simulink model "WF_onshore"  (R2024a)
settings: Solver=VariableStepAuto  StartTime=0  StopTime=0.9  RelTol=1e-3
values from neighbouring files (symbols this model uses):
  cvtr = initialize_NR_VSC_GF(cvtr)    [NR_steadystate_VSC_GF.m]    (also in WF_onshore_SSO_GFL.m = setfield(cvtr,'parameters', p_vary.name,p_vary.val(i)); WF_physical_param_offshore_supersynchronous.m = setfield(cvtr,'parameters', p_vary.name,p_vary.val(i)); WF_physical_param_onshore_SSO_020625.m = setfield(cvtr,'parameters', p_vary.name,p_vary.val(i)); impedance_WT_blackbox.m = base_values(cvtr))
  cvtr1 = cvtr_agg    [WF_physical_param_onshore_SSO_020625.m]
  enable_pll = 1    [impedance_WT_agg.m]    (also in initialize_WT_agg.m; initialize_WT_default_gfl.m; initialize_WT_default_offshore_super.m)
  f1 = 50    [WF_onshore_SSO_GFL.m]    (also in WF_physical_param_offshore_supersynchronous.m; WF_physical_param_onshore_SSO_020625.m; initialize_params_agg.m)
  i = 1    [WF_physical_param_offshore_supersynchronous.m]    (also in WF_physical_param_onshore_SSO_020625.m)
  L = inv(R)    [participation_factors_VSC_GF.m]
  l_OH = 0.2    [WF_onshore_SSO_GFL.m]    (also in WF_physical_param_offshore_supersynchronous.m = 0.1; WF_physical_param_onshore_SSO_020625.m = 0.1; initialize_params_agg.m = 0.1)
  l_tf_wf = tf_params(2,2)    [IM_WF_agg.m]    (also in WF_onshore_SSO_GFL.m = 0.05; WF_physical_param_offshore_supersynchronous.m = 0.05; WF_physical_param_onshore_SSO_020625.m = 0.05; initialize_params_agg.m = 0.05)
  l_tf_wt = tf_params(1,2)    [IM_WF_agg.m]    (also in WF_onshore_SSO_GFL.m = 0.0392; WF_physical_param_offshore_supersynchronous.m = 0.0392; WF_physical_param_onshore_SSO_020625.m = 0.0392; initialize_params_agg.m = 0.0392)
  Lg = p_vary(i)*((Z_b_G/(2*pi*f1)))    [WF_onshore_SSO_GFL.m]    (also in WF_physical_param_offshore_supersynchronous.m; WF_physical_param_onshore_SSO_020625.m; initialize_params_agg.m = 0.1*((Z_b_G/(2*pi*f1))))
  Lg1 = Lg    [WF_physical_param_offshore_supersynchronous.m]    (also in WF_physical_param_onshore_SSO_020625.m)
  Lg2 = Lg    [WF_physical_param_offshore_supersynchronous.m]    (also in WF_physical_param_onshore_SSO_020625.m)
  r_OH = 0.02    [WF_onshore_SSO_GFL.m]    (also in WF_physical_param_offshore_supersynchronous.m = 0.01; WF_physical_param_onshore_SSO_020625.m = 0.01; initialize_params_agg.m)
  r_tf_wf = tf_params(2,1)    [IM_WF_agg.m]    (also in WF_onshore_SSO_GFL.m = 0.005; WF_physical_param_offshore_supersynchronous.m = 0.005; WF_physical_param_onshore_SSO_020625.m = 0.005; initialize_params_agg.m = 0.005)
  r_tf_wt = tf_params(1,1)    [IM_WF_agg.m]    (also in WF_onshore_SSO_GFL.m = 0.0056; WF_physical_param_offshore_supersynchronous.m = 0.0056; WF_physical_param_onshore_SSO_020625.m = 0.0056; initialize_params_agg.m = 0.0056)
  Rg = rg*Z_b_G    [WF_onshore_SSO_GFL.m]    (also in WF_physical_param_offshore_supersynchronous.m; WF_physical_param_onshore_SSO_020625.m; initialize_params_agg.m = 0.01*Z_b_G)
  Sb_WF = (3*1)*5e6    (= 15000000)    [WF_onshore_SSO_GFL.m]    (also in WF_physical_param_offshore_supersynchronous.m; WF_physical_param_onshore_SSO_020625.m; impedance_WT_blackbox.m = n_t*Sb_WT; initialize_params_agg.m = 1000000000)
  Sb_WT = 5e6    (= 5000000)    [IM_WF.m]    (also in WF_onshore_SSO_GFL.m; WF_physical_param_offshore_supersynchronous.m; WF_physical_param_onshore_SSO_020625.m; initialize_params_agg.m)
  selector_current_reference = 3    [impedance_WT_agg.m]    (also in initialize_WT_agg.m; initialize_WT_default_gfl.m; initialize_WT_default_offshore_super.m)
  selector_omega_reference = 1    [impedance_WT_agg.m]    (also in initialize_WT_agg.m; initialize_WT_default_gfl.m; initialize_WT_default_offshore_super.m)
  V_coll = 33e3    (= 33000)    [WF_onshore_SSO_GFL.m]    (also in WF_physical_param_offshore_supersynchronous.m; WF_physical_param_onshore_SSO_020625.m; initialize_params_agg.m)
  V_trans = 220e3    (= 220000)    [WF_onshore_SSO_GFL.m]    (also in WF_physical_param_offshore_supersynchronous.m; WF_physical_param_onshore_SSO_020625.m; initialize_params_agg.m)
  Z_b_G = (V_trans/sqrt(3/2))^2/Sb_WF    [WF_onshore_SSO_GFL.m]    (also in WF_physical_param_offshore_supersynchronous.m = (V_b_trans)^2/Sb_WF; WF_physical_param_onshore_SSO_020625.m = (V_b_trans)^2/Sb_WF; initialize_params_agg.m = (V_b_trans)^2/Sb_WF)
undefined symbols (not defined in the file or in its folder): opts, R
libraries: simulink_extras x104, spsSeriesRLCBranchLib x90, simulink x52, spsThreePhaseVIMeasurementLib x42, spsControlledVoltageSourceLib x42, spsGroundLib x27, spsThreePhaseTransformerTwoWindingsLib x14, powerlib_extras x13, spsVariableInductorLib x6, spsPower3phInstantaneousLib x3, spspowerguiLib x1
(part 3 of 12)

== system WF_onshore/VoltageSource/grid inductance1 ==
  Rate Limiter : RateLimiter  SampleTimeMode=inherited
  Series RLC Branch : spsSeriesRLCBranchLib/Series RLC Branch  LConnTagsString=__new0  RConnTagsString=__new0  BranchType=R  Resistance=Rg+r_OH*Z_b_G  Inductance=Lg  SetiL0=off  InitialCurrent=cvtr.ss.io0a  Capacitance=1e-6  Setx0=off  InitialVoltage=0  Measurements=None
  Series RLC Branch1 : spsSeriesRLCBranchLib/Series RLC Branch  LConnTagsString=__new0  RConnTagsString=__new0  BranchType=R  Resistance=Rg+r_OH*Z_b_G  Inductance=Lg  SetiL0=off  InitialCurrent=cvtr.ss.io0b  Capacitance=1e-6  Setx0=off  InitialVoltage=0  Measurements=None
  Series RLC Branch2 : spsSeriesRLCBranchLib/Series RLC Branch  LConnTagsString=__new0  RConnTagsString=__new0  BranchType=R  Resistance=Rg+r_OH*Z_b_G  Inductance=Lg  SetiL0=off  InitialCurrent=cvtr.ss.io0c  Capacitance=1e-6  Setx0=off  InitialVoltage=0  Measurements=None
  Series RLC Branch3 : spsSeriesRLCBranchLib/Series RLC Branch  LConnTagsString=__new0  RConnTagsString=__new0  BranchType=R  Resistance=1e9  Inductance=Lg  SetiL0=off  InitialCurrent=cvtr.ss.io0a  Capacitance=1e-6  Setx0=off  InitialVoltage=0  Measurements=None
  Series RLC Branch4 : spsSeriesRLCBranchLib/Series RLC Branch  LConnTagsString=__new0  RConnTagsString=__new0  BranchType=R  Resistance=1e9  Inductance=Lg  SetiL0=off  InitialCurrent=cvtr.ss.io0a  Capacitance=1e-6  Setx0=off  InitialVoltage=0  Measurements=None
  Series RLC Branch5 : spsSeriesRLCBranchLib/Series RLC Branch  LConnTagsString=__new0  RConnTagsString=__new0  BranchType=R  Resistance=1e9  Inductance=Lg  SetiL0=off  InitialCurrent=cvtr.ss.io0a  Capacitance=1e-6  Setx0=off  InitialVoltage=0  Measurements=None
  Step : Step  Time=0.2  Before=(Lg1+l_OH*(Z_b_G/(2*pi*f1)))  After=(Lg2+l_OH*(Z_b_G/(2*pi*f1)))  SampleTime=0
  Variable Inductor : spsVariableInductorLib/Variable Inductor  methode=Backward Euler  Labsmin=1e-6  Initialize=off  iL0=0  L0=1e-3  Vl0=0
      settings: LibrarySourceBlock=sps_lib/Passives/Variable Inductor
  Variable Inductor1 : spsVariableInductorLib/Variable Inductor  methode=Backward Euler  Labsmin=1e-6  Initialize=off  iL0=0  L0=1e-3  Vl0=0
      settings: LibrarySourceBlock=sps_lib/Passives/Variable Inductor
  Variable Inductor2 : spsVariableInductorLib/Variable Inductor  methode=Backward Euler  Labsmin=1e-6  Initialize=off  iL0=0  L0=1e-3  Vl0=0
      settings: LibrarySourceBlock=sps_lib/Passives/Variable Inductor
  A : PMIOPort  Side=Left
  a : PMIOPort  Port=2  Side=Right
  B : PMIOPort  Port=3  Side=Left
  b : PMIOPort  Port=4  Side=Right
  C : PMIOPort  Port=5  Side=Left
  c : PMIOPort  Port=6  Side=Right
  wires:
  Step/1 -> Rate Limiter/1
  Rate Limiter/1 -> Variable Inductor2/1, Variable Inductor1/1, Variable Inductor/1
  connections:
  Series RLC Branch2/RConn1 -- c/RConn1
  Series RLC Branch1/RConn1 -- b/RConn1
  Series RLC Branch/RConn1 -- a/RConn1
  Series RLC Branch/LConn1 -- Series RLC Branch5/RConn1 -- Variable Inductor/RConn1
  Series RLC Branch1/LConn1 -- Series RLC Branch4/RConn1 -- Variable Inductor1/RConn1
  Series RLC Branch2/LConn1 -- Series RLC Branch3/RConn1 -- Variable Inductor2/RConn1
  A/RConn1 -- Series RLC Branch5/LConn1 -- Variable Inductor/LConn1
  B/RConn1 -- Series RLC Branch4/LConn1 -- Variable Inductor1/LConn1
  C/RConn1 -- Series RLC Branch3/LConn1 -- Variable Inductor2/LConn1

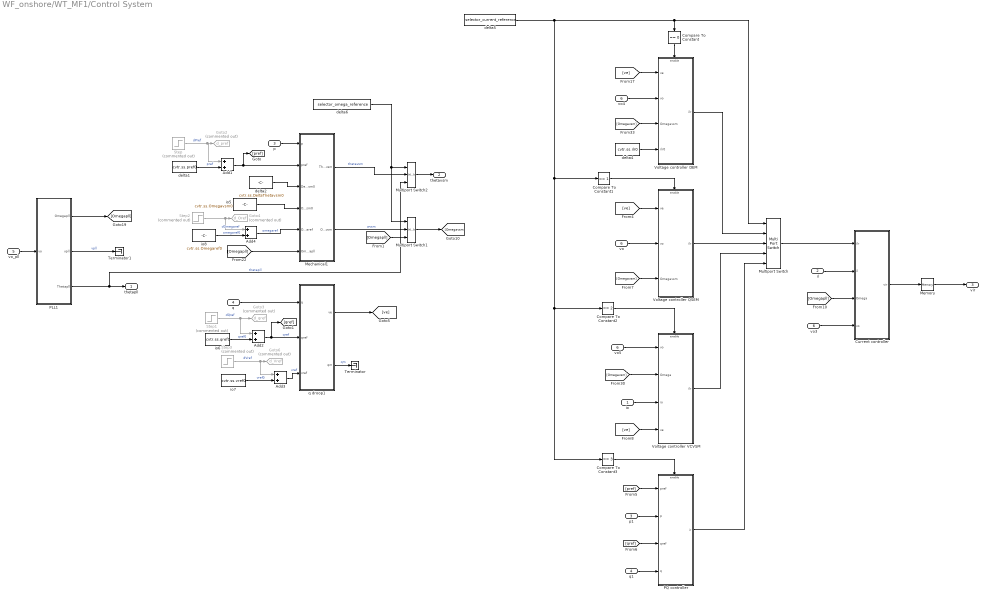
== system WF_onshore/WT_MF1/Control System ==
  io : Inport
  il : Inport  Port=2
  p : Inport  Port=3
  q : Inport  Port=4
  vo_pll : Inport  Port=5
  vo : Inport  Port=6
  Add{1..4} (4 alike) : Sum
  Compare To Constant : simulink/Logic and Bit Operations/Compare To Constant  relop===  const=0  OutDataTypeStr=boolean
  Compare To Constant1 : simulink/Logic and Bit Operations/Compare To Constant  relop===  const=1  OutDataTypeStr=boolean
  Compare To Constant2 : simulink/Logic and Bit Operations/Compare To Constant  relop===  const=2  OutDataTypeStr=boolean
  Compare To Constant3 : simulink/Logic and Bit Operations/Compare To Constant  relop===  const=3  OutDataTypeStr=boolean
  Current controller : Subsystem
  Goto2 : Goto  Commented=on  GotoTag=d_pref  TagVisibility=global
  Goto3 : Goto  Commented=on  GotoTag=d_qref  TagVisibility=global
  Goto4 : Goto  Commented=on  GotoTag=d_Oref  TagVisibility=global
  Goto6 : Goto  Commented=on  GotoTag=d_Vref  TagVisibility=global
  Mechanical1 : Subsystem
  Memory : Memory  InitialCondition=cvtr.ss.vir0
  Multiport Switch : MultiPortSwitch  DataPortOrder=Zero-based contiguous  Inputs=4  zeroidx=on  SaturateOnIntegerOverflow=off  InputSameDT=off
  Multiport Switch1 : MultiPortSwitch  DataPortOrder=Zero-based contiguous  Inputs=2  zeroidx=on  SaturateOnIntegerOverflow=off  InputSameDT=off
  Multiport Switch2 : MultiPortSwitch  DataPortOrder=Zero-based contiguous  Inputs=2  zeroidx=on  SaturateOnIntegerOverflow=off  InputSameDT=off
  PLL1 : Subsystem
  PQ controller : Subsystem
  Step : Step  Commented=on  After=0.01  SampleTime=0
  Step1 : Step  Commented=on  Time=1.5  After=0.03  SampleTime=0
  Step2 : Step  Commented=on  Time=2  After=0.001  SampleTime=0
  Step3 : Step  Commented=on  Time=2  After=0.001  SampleTime=0
  Terminator : Terminator
  Terminator1 : Terminator
  Voltage controller DEM : Subsystem
  Voltage controller QSEM : Subsystem
  Voltage controller VCVSM : Subsystem
  delta1 : Constant  Value=cvtr.ss.pref0
  delta2 : Constant  Value=cvtr.ss.DeltaThetavsm0
  delta4 : Constant  Value=cvtr.ss.ilr0
  delta5 : Constant  Value=selector_current_reference
  delta6 : Constant  Value=selector_omega_reference
  io5 : Constant  Value=cvtr.ss.Omegavsm0
  io6 : Constant  Value=cvtr.ss.qref0
  io7 : Constant  Value=cvtr.ss.vref0
  io8 : Constant  Value=cvtr.ss.Omegaref0
  p1 : InportShadow  Port=3
  q droop1 : Subsystem
  q1 : InportShadow  Port=4
  vo3 : InportShadow  Port=6
  vo4 : InportShadow  Port=6
  vo5 : InportShadow  Port=6
  thetapll : Outport
  thetavsm : Outport  Port=2
  vir : Outport  Port=3
  wires:
  io5/1 -> Mechanical1/4(Omegavsm0)
  Voltage controller DEM/1(ilr) -> Multiport Switch/2
  Add1/1 -> [pref], Mechanical1/2(pref)
  delta4/1 -> Voltage controller DEM/4(ilr0)
  Multiport Switch/1 -> Current controller/1(ilr)
  delta2/1 -> Mechanical1/3(DeltaThetavsm0)
  Add2/1 -> [qref], q droop1/2(qref)  "qref"
  delta1/1 -> Add1/2  "pref"
  q droop1/2(qm) -> Terminator/1  "qm"
  Add4/1 -> Mechanical1/5(Omegaref)  "omegaref"
  io7/1 -> Add3/2  "vref0"
  [Omegavsm] -> Voltage controller QSEM/3(Omegavsm)
  io8/1 -> Add4/2  "omegaref0"
  Step/1 -> Add1/1, Goto2/1  "dPref"
  [ve] -> Voltage controller QSEM/1(ve)
  delta5/1 -> Compare To Constant3/1, Compare To Constant2/1, Compare To Constant1/1, Multiport Switch/1, Compare To Constant/1
  io6/1 -> Add2/2  "qref0"
  Add3/1 -> q droop1/3(vref)  "vref"
  q/1 -> q droop1/1(q)
  [Omegavsm] -> Voltage controller VCVSM/2(Omega)
  [ve] -> Voltage controller DEM/1(ve)
  [Omegapll] -> Mechanical1/6(Omegapll)
  [Omegavsm] -> Voltage controller DEM/3(Omegavsm)
  p/1 -> Mechanical1/1(p)
  Voltage controller VCVSM/1(ilr) -> Multiport Switch/4
  vo/1 -> Voltage controller QSEM/2(vo)
  vo_pll/1 -> PLL1/1(vo)
  PLL1/2(vpll) -> Terminator1/1  "vpll"
  q droop1/1(ve) -> [ve]
  Voltage controller QSEM/1(ilr) -> Multiport Switch/3
  Memory/1 -> vir/1
  Current controller/1(vir) -> Memory/1
  p1/1 -> PQ controller/2(p)
  q1/1 -> PQ controller/4(q)
  PQ controller/1(ir) -> Multiport Switch/5
  il/1 -> Current controller/2(il)
  delta6/1 -> Multiport Switch2/1, Multiport Switch1/1
  [Omegapll] -> Current controller/3(Omega)
  Mechanical1/2(Omegavsm) -> Multiport Switch1/2  "wvsm"
  [Omegapll] -> Multiport Switch1/3
  Multiport Switch2/1 -> thetavsm/1
  Mechanical1/1(Thetavsm) -> Multiport Switch2/2  "thetavsm"
  Compare To Constant/1 -> Voltage controller DEM/Enable
  Compare To Constant1/1 -> Voltage controller QSEM/Enable
  Compare To Constant2/1 -> Voltage controller VCVSM/Enable
  Compare To Constant3/1 -> PQ controller/Enable
  Multiport Switch1/1 -> [Omegavsm]
  PLL1/1(Omegapll) -> [Omegapll]
  PLL1/3(Thetapll) -> Multiport Switch2/3, thetapll/1  "thetapll"
  io/1 -> Voltage controller VCVSM/3(io)
  vo3/1 -> Current controller/4(vo)
  vo4/1 -> Voltage controller DEM/2(vo)
  vo5/1 -> Voltage controller VCVSM/1(vo)
  [ve] -> Voltage controller VCVSM/4(ve)
  [pref] -> PQ controller/1(pref)
  [qref] -> PQ controller/3(qref)
  Step1/1 -> Goto3/1, Add2/1  "dQref"
  Step2/1 -> Add4/1, Goto4/1  "dOmegaref"
  Step3/1 -> Add3/1, Goto6/1  "dVref"

== system WF_onshore/WT_MF1/Inverse Park1 ==
  x_dq : Inport
  delta : Inport  Port=2
  Demux1 : Demux  Outputs=2
  Fcn : Fcn  Expr=cos(u(3))*u(1)-sin(u(3))*u(2)
  Fcn1 : Fcn  Expr=cos(u(3)-2/3*pi)*u(1)-sin(u(3)-2/3*pi)*u(2)
  Fcn2 : Fcn  Expr=cos(u(3)+2/3*pi)*u(1)-sin(u(3)+2/3*pi)*u(2)
  Mux : Mux  Inputs=3
  Mux1 : Mux  Inputs=3
  x_abc : Outport
  wires:
  Mux/1 -> Fcn1/1, Fcn2/1, Fcn/1
  Demux1/2 -> Mux/2
  Demux1/1 -> Mux/1
  Fcn/1 -> Mux1/1
  Fcn1/1 -> Mux1/2
  Fcn2/1 -> Mux1/3
  Mux1/1 -> x_abc/1
  x_dq/1 -> Demux1/1
  delta/1 -> Mux/3

== system WF_onshore/WT_MF1/Subsystem1 ==
  v_abc : Inport
  Controlled Voltage Source : spsControlledVoltageSourceLib/Controlled Voltage Source  Initialize=on  Source_Type=AC  Amplitude=0  Phase=0  Frequency=0  Measurements=None
  Controlled Voltage Source1 : spsControlledVoltageSourceLib/Controlled Voltage Source  Initialize=on  Source_Type=AC  Amplitude=0  Phase=0  Frequency=0  Measurements=None
  Controlled Voltage Source2 : spsControlledVoltageSourceLib/Controlled Voltage Source  Initialize=on  Source_Type=AC  Amplitude=0  Phase=0  Frequency=0  Measurements=None
  Demux : Demux  Outputs=3
  Ground : spsGroundLib/Ground  LConnTagsString=a
  va1 : PMIOPort  Side=Right
  vb1 : PMIOPort  Port=2  Side=Right
  vc1 : PMIOPort  Port=3  Side=Right
  wires:
  v_abc/1 -> Demux/1
  Demux/3 -> Controlled Voltage Source2/1
  Demux/2 -> Controlled Voltage Source1/1
  Demux/1 -> Controlled Voltage Source/1
  connections:
  Controlled Voltage Source/LConn1 -- Controlled Voltage Source1/LConn1 -- Controlled Voltage Source2/LConn1 -- Ground/LConn1
  vc1/RConn1 -- Controlled Voltage Source2/RConn1
  vb1/RConn1 -- Controlled Voltage Source1/RConn1
  va1/RConn1 -- Controlled Voltage Source/RConn1

== system WF_onshore/WT_MF1/Subsystem6 ==
  x_d+ix_q : Inport
  Complex to Real-Imag2 : ComplexToRealImag
  Mux : Mux  Inputs=2
  x_dq : Outport
  wires:
  Complex to Real-Imag2/1 -> Mux/1
  Complex to Real-Imag2/2 -> Mux/2
  Mux/1 -> x_dq/1
  x_d+ix_q/1 -> Complex to Real-Imag2/1

== system WF_onshore/WT_MF1/Transformations (pu and dq) ==
  i_abc_grid : Inport
  i_abc_filt : Inport  Port=2
  v_abc_grid : Inport  Port=3
  v_abc_filt : Inport  Port=4
  Thetavsm : Inport  Port=5
  Thetapll : Inport  Port=6
  3-phase Instantaneous Active & Reactive Power : powerlib_extras/Measurements/3-phase  Instantaneous  Active & Reactive Power
  Demux : Demux  Outputs=2
  Gain : Gain  Gain=1/cvtr.pu.Vb
  Gain1 : Gain  Gain=1/cvtr.pu.Ib
  Gain2 : Gain  Gain=1/cvtr.pu.Sb
  Gain4 : Gain  Gain=1/cvtr.pu.Ib
  Gain6 : Gain  Gain=1/cvtr.pu.Vb
  I_conv : ToWorkspace  VariableName=I_dq  SaveFormat=Structure With Time  SampleTime=-1
      settings: MaxDataPoints=1000000
  Park : Subsystem
  Park1 : Subsystem
  Park2 : Subsystem
  Park4 : Subsystem
  Scope{,1..2,4} (4 alike) : Scope  Commented=on
  Scope3 : Scope  Commented=on  NumInputPorts=2
  Subsystem2 : Subsystem
  Subsystem3 : Subsystem
  Subsystem4 : Subsystem
  Subsystem7 : Subsystem
  V_conv : ToWorkspace  VariableName=V_dq  SaveFormat=Structure With Time  SampleTime=-1
      settings: MaxDataPoints=1000000
  io : Outport
  il : Outport  Port=2
  p : Outport  Port=3
  q : Outport  Port=4
  vo_pll : Outport  Port=5
  vo : Outport  Port=6
  wires:
  Gain6/1 -> Park4/1(x_abc)
  i_abc_grid/1 -> 3-phase Instantaneous Active & Reactive Power/2, Gain1/1
  Gain2/1 -> Demux/1
  Gain1/1 -> Park1/1(x_abc)
  Gain/1 -> Park2/1(x_abc)
  Gain4/1 -> Park/1(x_abc)
  Park4/1(x_dq) -> Subsystem2/1(x_dq)
  Demux/1 -> Scope3/1, p/1
  i_abc_filt/1 -> Gain4/1
  Thetapll/1 -> Park4/2(delta)
  Subsystem2/1(x_d+ix_q) -> Scope4/1, vo_pll/1
  Thetavsm/1 -> Park1/2(delta), Park2/2(delta), Park/2(delta)
  Demux/2 -> Scope3/2, q/1
  v_abc_grid/1 -> 3-phase Instantaneous Active & Reactive Power/1
  3-phase Instantaneous Active & Reactive Power/1 -> Gain2/1
  Subsystem4/1(x_d+ix_q) -> io/1
  Subsystem7/1(x_d+ix_q) -> il/1, Scope/1
  Subsystem3/1(x_d+ix_q) -> vo/1
  Park/1(x_dq) -> Subsystem7/1(x_dq)
  Park1/1(x_dq) -> I_conv/1, Scope2/1, Subsystem4/1(x_dq)
  Park2/1(x_dq) -> V_conv/1, Scope1/1, Subsystem3/1(x_dq)
  v_abc_filt/1 -> Gain/1, Gain6/1

== system WF_onshore/WT_MF1/filter capacitance1 ==
  Ground : spsGroundLib/Ground  LConnTagsString=a
  Series RLC Branch : spsSeriesRLCBranchLib/Series RLC Branch  LConnTagsString=__new0  RConnTagsString=__new0  BranchType=C  Resistance=R  Inductance=L  SetiL0=on  InitialCurrent=ia0  Capacitance=cvtr.parameters.Cf  Setx0=on  InitialVoltage=cvtr.ss.vo0a  Measurements=None
  Series RLC Branch1 : spsSeriesRLCBranchLib/Series RLC Branch  LConnTagsString=__new0  RConnTagsString=__new0  BranchType=C  Resistance=R  Inductance=L  SetiL0=on  InitialCurrent=ia0  Capacitance=cvtr.parameters.Cf  Setx0=on  InitialVoltage=cvtr.ss.vo0b  Measurements=None
  Series RLC Branch2 : spsSeriesRLCBranchLib/Series RLC Branch  LConnTagsString=__new0  RConnTagsString=__new0  BranchType=C  Resistance=R  Inductance=L  SetiL0=on  InitialCurrent=ia0  Capacitance=cvtr.parameters.Cf  Setx0=on  InitialVoltage=cvtr.ss.vo0c  Measurements=None
  Three-Phase V-I Measurement : spsThreePhaseVIMeasurementLib/Three-Phase V-I Measurement  VoltageMeasurement=phase-to-ground  SetLabelV=off  LabelV=Vabc  Vpu=off  VpuLL=off  CurrentMeasurement=no  SetLabelI=off  LabelI=Iabc  Ipu=off  Pbase=100e6  Vbase=500e3  OutputType=Complex  PhasorSimulation=off  PSBequivalent=0
  A : PMIOPort  Side=Left
  B : PMIOPort  Port=2  Side=Left
  C : PMIOPort  Port=3  Side=Left
  v_abc : Outport
  wires:
  Three-Phase V-I Measurement/1 -> v_abc/1
  connections:
  A/RConn1 -- Three-Phase V-I Measurement/LConn1
  B/RConn1 -- Three-Phase V-I Measurement/LConn2
  C/RConn1 -- Three-Phase V-I Measurement/LConn3
  Three-Phase V-I Measurement/RConn1 -- Series RLC Branch/LConn1
  Three-Phase V-I Measurement/RConn2 -- Series RLC Branch1/LConn1
  Three-Phase V-I Measurement/RConn3 -- Series RLC Branch2/LConn1
  Series RLC Branch/RConn1 -- Ground/LConn1 -- Series RLC Branch1/RConn1 -- Series RLC Branch2/RConn1

== system WF_onshore/WT_MF1/filter inductance1 ==
  Series RLC Branch : spsSeriesRLCBranchLib/Series RLC Branch  LConnTagsString=__new0  RConnTagsString=__new0  BranchType=RL  Resistance=cvtr.parameters.Rf  Inductance=cvtr.parameters.Lf  SetiL0=on  InitialCurrent=cvtr.ss.il0a  Capacitance=1e-6  Setx0=off  InitialVoltage=0  Measurements=None
  Series RLC Branch1 : spsSeriesRLCBranchLib/Series RLC Branch  LConnTagsString=__new0  RConnTagsString=__new0  BranchType=RL  Resistance=cvtr.parameters.Rf  Inductance=cvtr.parameters.Lf  SetiL0=on  InitialCurrent=cvtr.ss.il0b  Capacitance=1e-6  Setx0=off  InitialVoltage=0  Measurements=None
  Series RLC Branch2 : spsSeriesRLCBranchLib/Series RLC Branch  LConnTagsString=__new0  RConnTagsString=__new0  BranchType=RL  Resistance=cvtr.parameters.Rf  Inductance=cvtr.parameters.Lf  SetiL0=on  InitialCurrent=cvtr.ss.il0c  Capacitance=1e-6  Setx0=off  InitialVoltage=0  Measurements=None
  Three-Phase V-I Measurement : spsThreePhaseVIMeasurementLib/Three-Phase V-I Measurement  VoltageMeasurement=no  SetLabelV=off  LabelV=Vabc  Vpu=off  VpuLL=off  CurrentMeasurement=yes  SetLabelI=off  LabelI=Iabc  Ipu=off  Pbase=100e6  Vbase=500e3  OutputType=Complex  PhasorSimulation=off  PSBequivalent=0
  A : PMIOPort  Side=Left
  B : PMIOPort  Port=2  Side=Left
  C : PMIOPort  Port=3  Side=Left
  a : PMIOPort  Port=4  Side=Right
  b : PMIOPort  Port=5  Side=Right
  c : PMIOPort  Port=6  Side=Right
  i_abc : Outport
  wires:
  Three-Phase V-I Measurement/1 -> i_abc/1
  connections:
  c/RConn1 -- Three-Phase V-I Measurement/RConn3
  C/RConn1 -- Series RLC Branch2/LConn1
  b/RConn1 -- Three-Phase V-I Measurement/RConn2
  B/RConn1 -- Series RLC Branch1/LConn1
  a/RConn1 -- Three-Phase V-I Measurement/RConn1
  A/RConn1 -- Series RLC Branch/LConn1
  Series RLC Branch2/RConn1 -- Three-Phase V-I Measurement/LConn3
  Series RLC Branch1/RConn1 -- Three-Phase V-I Measurement/LConn2
  Series RLC Branch/RConn1 -- Three-Phase V-I Measurement/LConn1

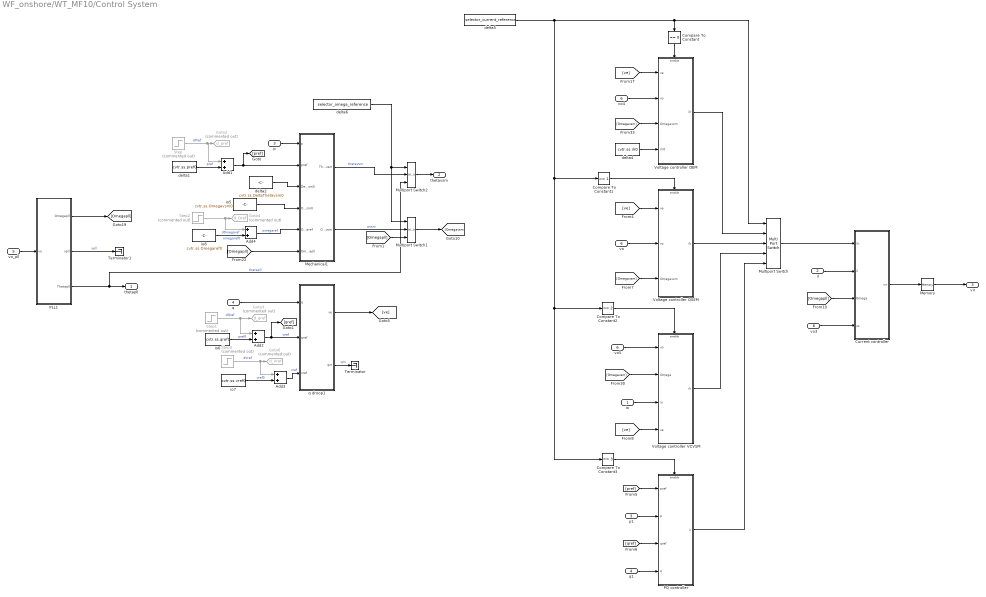
== system WF_onshore/WT_MF10/Control System ==
  io : Inport
  il : Inport  Port=2
  p : Inport  Port=3
  q : Inport  Port=4
  vo_pll : Inport  Port=5
  vo : Inport  Port=6
  Add{1..4} (4 alike) : Sum
  Compare To Constant : simulink/Logic and Bit Operations/Compare To Constant  relop===  const=0  OutDataTypeStr=boolean
  Compare To Constant1 : simulink/Logic and Bit Operations/Compare To Constant  relop===  const=1  OutDataTypeStr=boolean
  Compare To Constant2 : simulink/Logic and Bit Operations/Compare To Constant  relop===  const=2  OutDataTypeStr=boolean
  Compare To Constant3 : simulink/Logic and Bit Operations/Compare To Constant  relop===  const=3  OutDataTypeStr=boolean
  Current controller : Subsystem
  Goto2 : Goto  Commented=on  GotoTag=d_pref  TagVisibility=global
  Goto3 : Goto  Commented=on  GotoTag=d_qref  TagVisibility=global
  Goto4 : Goto  Commented=on  GotoTag=d_Oref  TagVisibility=global
  Goto6 : Goto  Commented=on  GotoTag=d_Vref  TagVisibility=global
  Mechanical1 : Subsystem
  Memory : Memory  InitialCondition=cvtr.ss.vir0
  Multiport Switch : MultiPortSwitch  DataPortOrder=Zero-based contiguous  Inputs=4  zeroidx=on  SaturateOnIntegerOverflow=off  InputSameDT=off
  Multiport Switch1 : MultiPortSwitch  DataPortOrder=Zero-based contiguous  Inputs=2  zeroidx=on  SaturateOnIntegerOverflow=off  InputSameDT=off
  Multiport Switch2 : MultiPortSwitch  DataPortOrder=Zero-based contiguous  Inputs=2  zeroidx=on  SaturateOnIntegerOverflow=off  InputSameDT=off
  PLL1 : Subsystem
  PQ controller : Subsystem
  Step : Step  Commented=on  After=0.01  SampleTime=0
  Step1 : Step  Commented=on  Time=1.5  After=0.03  SampleTime=0
  Step2 : Step  Commented=on  Time=2  After=0.001  SampleTime=0
  Step3 : Step  Commented=on  Time=2  After=0.001  SampleTime=0
  Terminator : Terminator
  Terminator1 : Terminator
  Voltage controller DEM : Subsystem
  Voltage controller QSEM : Subsystem
  Voltage controller VCVSM : Subsystem
  delta1 : Constant  Value=cvtr.ss.pref0
  delta2 : Constant  Value=cvtr.ss.DeltaThetavsm0
  delta4 : Constant  Value=cvtr.ss.ilr0
  delta5 : Constant  Value=selector_current_reference
  delta6 : Constant  Value=selector_omega_reference
  io5 : Constant  Value=cvtr.ss.Omegavsm0
  io6 : Constant  Value=cvtr.ss.qref0
  io7 : Constant  Value=cvtr.ss.vref0
  io8 : Constant  Value=cvtr.ss.Omegaref0
  p1 : InportShadow  Port=3
  q droop1 : Subsystem
  q1 : InportShadow  Port=4
  vo3 : InportShadow  Port=6
  vo4 : InportShadow  Port=6
  vo5 : InportShadow  Port=6
  thetapll : Outport
  thetavsm : Outport  Port=2
  vir : Outport  Port=3
  wires:
  Step3/1 -> Goto6/1, Add3/1  "dVref"
  Step2/1 -> Goto4/1, Add4/1  "dOmegaref"
  Step1/1 -> Add2/1, Goto3/1  "dQref"
  [qref] -> PQ controller/3(qref)
  [pref] -> PQ controller/1(pref)
  [ve] -> Voltage controller VCVSM/4(ve)
  vo5/1 -> Voltage controller VCVSM/1(vo)
  vo4/1 -> Voltage controller DEM/2(vo)
  vo3/1 -> Current controller/4(vo)
  io/1 -> Voltage controller VCVSM/3(io)
  PLL1/3(Thetapll) -> thetapll/1, Multiport Switch2/3  "thetapll"
  PLL1/1(Omegapll) -> [Omegapll]
  Multiport Switch1/1 -> [Omegavsm]
  Compare To Constant3/1 -> PQ controller/Enable
  Compare To Constant2/1 -> Voltage controller VCVSM/Enable
  Compare To Constant1/1 -> Voltage controller QSEM/Enable
  Compare To Constant/1 -> Voltage controller DEM/Enable
  Mechanical1/1(Thetavsm) -> Multiport Switch2/2  "thetavsm"
  Multiport Switch2/1 -> thetavsm/1
  [Omegapll] -> Multiport Switch1/3
  Mechanical1/2(Omegavsm) -> Multiport Switch1/2  "wvsm"
  [Omegapll] -> Current controller/3(Omega)
  delta6/1 -> Multiport Switch1/1, Multiport Switch2/1
  il/1 -> Current controller/2(il)
  PQ controller/1(ir) -> Multiport Switch/5
  q1/1 -> PQ controller/4(q)
  p1/1 -> PQ controller/2(p)
  Current controller/1(vir) -> Memory/1
  Memory/1 -> vir/1
  Voltage controller QSEM/1(ilr) -> Multiport Switch/3
  q droop1/1(ve) -> [ve]
  PLL1/2(vpll) -> Terminator1/1  "vpll"
  vo_pll/1 -> PLL1/1(vo)
  vo/1 -> Voltage controller QSEM/2(vo)
  Voltage controller VCVSM/1(ilr) -> Multiport Switch/4
  p/1 -> Mechanical1/1(p)
  [Omegavsm] -> Voltage controller DEM/3(Omegavsm)
  [Omegapll] -> Mechanical1/6(Omegapll)
  [ve] -> Voltage controller DEM/1(ve)
  [Omegavsm] -> Voltage controller VCVSM/2(Omega)
  q/1 -> q droop1/1(q)
  Add3/1 -> q droop1/3(vref)  "vref"
  io6/1 -> Add2/2  "qref0"
  delta5/1 -> Compare To Constant/1, Multiport Switch/1, Compare To Constant1/1, Compare To Constant2/1, Compare To Constant3/1
  [ve] -> Voltage controller QSEM/1(ve)
  Step/1 -> Goto2/1, Add1/1  "dPref"
  io8/1 -> Add4/2  "omegaref0"
  [Omegavsm] -> Voltage controller QSEM/3(Omegavsm)
  io7/1 -> Add3/2  "vref0"
  Add4/1 -> Mechanical1/5(Omegaref)  "omegaref"
  q droop1/2(qm) -> Terminator/1  "qm"
  delta1/1 -> Add1/2  "pref"
  Add2/1 -> q droop1/2(qref), [qref]  "qref"
  delta2/1 -> Mechanical1/3(DeltaThetavsm0)
  Multiport Switch/1 -> Current controller/1(ilr)
  delta4/1 -> Voltage controller DEM/4(ilr0)
  Add1/1 -> Mechanical1/2(pref), [pref]
  Voltage controller DEM/1(ilr) -> Multiport Switch/2
  io5/1 -> Mechanical1/4(Omegavsm0)

== system WF_onshore/WT_MF10/Inverse Park1 ==
  x_dq : Inport
  delta : Inport  Port=2
  Demux1 : Demux  Outputs=2
  Fcn : Fcn  Expr=cos(u(3))*u(1)-sin(u(3))*u(2)
  Fcn1 : Fcn  Expr=cos(u(3)-2/3*pi)*u(1)-sin(u(3)-2/3*pi)*u(2)
  Fcn2 : Fcn  Expr=cos(u(3)+2/3*pi)*u(1)-sin(u(3)+2/3*pi)*u(2)
  Mux : Mux  Inputs=3
  Mux1 : Mux  Inputs=3
  x_abc : Outport
  wires:
  delta/1 -> Mux/3
  x_dq/1 -> Demux1/1
  Mux1/1 -> x_abc/1
  Fcn2/1 -> Mux1/3
  Fcn1/1 -> Mux1/2
  Fcn/1 -> Mux1/1
  Demux1/1 -> Mux/1
  Demux1/2 -> Mux/2
  Mux/1 -> Fcn/1, Fcn2/1, Fcn1/1

== system WF_onshore/WT_MF10/Subsystem1 ==
  v_abc : Inport
  Controlled Voltage Source : spsControlledVoltageSourceLib/Controlled Voltage Source  Initialize=on  Source_Type=AC  Amplitude=0  Phase=0  Frequency=0  Measurements=None
  Controlled Voltage Source1 : spsControlledVoltageSourceLib/Controlled Voltage Source  Initialize=on  Source_Type=AC  Amplitude=0  Phase=0  Frequency=0  Measurements=None
  Controlled Voltage Source2 : spsControlledVoltageSourceLib/Controlled Voltage Source  Initialize=on  Source_Type=AC  Amplitude=0  Phase=0  Frequency=0  Measurements=None
  Demux : Demux  Outputs=3
  Ground : spsGroundLib/Ground  LConnTagsString=a
  va1 : PMIOPort  Side=Right
  vb1 : PMIOPort  Port=2  Side=Right
  vc1 : PMIOPort  Port=3  Side=Right
  wires:
  Demux/1 -> Controlled Voltage Source/1
  Demux/2 -> Controlled Voltage Source1/1
  Demux/3 -> Controlled Voltage Source2/1
  v_abc/1 -> Demux/1
  connections:
  va1/RConn1 -- Controlled Voltage Source/RConn1
  vb1/RConn1 -- Controlled Voltage Source1/RConn1
  vc1/RConn1 -- Controlled Voltage Source2/RConn1
  Ground/LConn1 -- Controlled Voltage Source2/LConn1 -- Controlled Voltage Source1/LConn1 -- Controlled Voltage Source/LConn1

== system WF_onshore/WT_MF10/Subsystem6 ==
  x_d+ix_q : Inport
  Complex to Real-Imag2 : ComplexToRealImag
  Mux : Mux  Inputs=2
  x_dq : Outport
  wires:
  x_d+ix_q/1 -> Complex to Real-Imag2/1
  Mux/1 -> x_dq/1
  Complex to Real-Imag2/2 -> Mux/2
  Complex to Real-Imag2/1 -> Mux/1

== system WF_onshore/WT_MF10/Transformations (pu and dq) ==
  i_abc_grid : Inport
  i_abc_filt : Inport  Port=2
  v_abc_grid : Inport  Port=3
  v_abc_filt : Inport  Port=4
  Thetavsm : Inport  Port=5
  Thetapll : Inport  Port=6
  3-phase Instantaneous Active & Reactive Power : powerlib_extras/Measurements/3-phase  Instantaneous  Active & Reactive Power
  Demux : Demux  Outputs=2
  Gain : Gain  Gain=1/cvtr.pu.Vb
  Gain1 : Gain  Gain=1/cvtr.pu.Ib
  Gain2 : Gain  Gain=1/cvtr.pu.Sb
  Gain4 : Gain  Gain=1/cvtr.pu.Ib
  Gain6 : Gain  Gain=1/cvtr.pu.Vb
  Park : Subsystem
  Park1 : Subsystem
  Park2 : Subsystem
  Park4 : Subsystem
  Subsystem2 : Subsystem
  Subsystem3 : Subsystem
  Subsystem4 : Subsystem
  Subsystem7 : Subsystem
  io : Outport
  il : Outport  Port=2
  p : Outport  Port=3
  q : Outport  Port=4
  vo_pll : Outport  Port=5
  vo : Outport  Port=6
  wires:
  v_abc_filt/1 -> Gain6/1, Gain/1
  Park2/1(x_dq) -> Subsystem3/1(x_dq)
  Park1/1(x_dq) -> Subsystem4/1(x_dq)
  Park/1(x_dq) -> Subsystem7/1(x_dq)
  Subsystem3/1(x_d+ix_q) -> vo/1
  Subsystem7/1(x_d+ix_q) -> il/1
  Subsystem4/1(x_d+ix_q) -> io/1
  3-phase Instantaneous Active & Reactive Power/1 -> Gain2/1
  v_abc_grid/1 -> 3-phase Instantaneous Active & Reactive Power/1
  Demux/2 -> q/1
  Thetavsm/1 -> Park/2(delta), Park2/2(delta), Park1/2(delta)
  Subsystem2/1(x_d+ix_q) -> vo_pll/1
  Thetapll/1 -> Park4/2(delta)
  i_abc_filt/1 -> Gain4/1
  Demux/1 -> p/1
  Park4/1(x_dq) -> Subsystem2/1(x_dq)
  Gain4/1 -> Park/1(x_abc)
  Gain/1 -> Park2/1(x_abc)
  Gain1/1 -> Park1/1(x_abc)
  Gain2/1 -> Demux/1
  i_abc_grid/1 -> Gain1/1, 3-phase Instantaneous Active & Reactive Power/2
  Gain6/1 -> Park4/1(x_abc)

== system WF_onshore/WT_MF10/filter capacitance1 ==
  Ground : spsGroundLib/Ground  LConnTagsString=a
  Series RLC Branch : spsSeriesRLCBranchLib/Series RLC Branch  LConnTagsString=__new0  RConnTagsString=__new0  BranchType=C  Resistance=R  Inductance=L  SetiL0=on  InitialCurrent=ia0  Capacitance=cvtr.parameters.Cf  Setx0=on  InitialVoltage=cvtr.ss.vo0a  Measurements=None
  Series RLC Branch1 : spsSeriesRLCBranchLib/Series RLC Branch  LConnTagsString=__new0  RConnTagsString=__new0  BranchType=C  Resistance=R  Inductance=L  SetiL0=on  InitialCurrent=ia0  Capacitance=cvtr.parameters.Cf  Setx0=on  InitialVoltage=cvtr.ss.vo0b  Measurements=None
  Series RLC Branch2 : spsSeriesRLCBranchLib/Series RLC Branch  LConnTagsString=__new0  RConnTagsString=__new0  BranchType=C  Resistance=R  Inductance=L  SetiL0=on  InitialCurrent=ia0  Capacitance=cvtr.parameters.Cf  Setx0=on  InitialVoltage=cvtr.ss.vo0c  Measurements=None
  Three-Phase V-I Measurement : spsThreePhaseVIMeasurementLib/Three-Phase V-I Measurement  VoltageMeasurement=phase-to-ground  SetLabelV=off  LabelV=Vabc  Vpu=off  VpuLL=off  CurrentMeasurement=no  SetLabelI=off  LabelI=Iabc  Ipu=off  Pbase=100e6  Vbase=500e3  OutputType=Complex  PhasorSimulation=off  PSBequivalent=0
  A : PMIOPort  Side=Left
  B : PMIOPort  Port=2  Side=Left
  C : PMIOPort  Port=3  Side=Left
  v_abc : Outport
  wires:
  Three-Phase V-I Measurement/1 -> v_abc/1
  connections:
  Series RLC Branch2/RConn1 -- Series RLC Branch1/RConn1 -- Ground/LConn1 -- Series RLC Branch/RConn1
  Three-Phase V-I Measurement/RConn3 -- Series RLC Branch2/LConn1
  Three-Phase V-I Measurement/RConn2 -- Series RLC Branch1/LConn1
  Three-Phase V-I Measurement/RConn1 -- Series RLC Branch/LConn1
  C/RConn1 -- Three-Phase V-I Measurement/LConn3
  B/RConn1 -- Three-Phase V-I Measurement/LConn2
  A/RConn1 -- Three-Phase V-I Measurement/LConn1

== system WF_onshore/WT_MF10/filter inductance1 ==
  Series RLC Branch : spsSeriesRLCBranchLib/Series RLC Branch  LConnTagsString=__new0  RConnTagsString=__new0  BranchType=RL  Resistance=cvtr.parameters.Rf  Inductance=cvtr.parameters.Lf  SetiL0=on  InitialCurrent=cvtr.ss.il0a  Capacitance=1e-6  Setx0=off  InitialVoltage=0  Measurements=None
  Series RLC Branch1 : spsSeriesRLCBranchLib/Series RLC Branch  LConnTagsString=__new0  RConnTagsString=__new0  BranchType=RL  Resistance=cvtr.parameters.Rf  Inductance=cvtr.parameters.Lf  SetiL0=on  InitialCurrent=cvtr.ss.il0b  Capacitance=1e-6  Setx0=off  InitialVoltage=0  Measurements=None
  Series RLC Branch2 : spsSeriesRLCBranchLib/Series RLC Branch  LConnTagsString=__new0  RConnTagsString=__new0  BranchType=RL  Resistance=cvtr.parameters.Rf  Inductance=cvtr.parameters.Lf  SetiL0=on  InitialCurrent=cvtr.ss.il0c  Capacitance=1e-6  Setx0=off  InitialVoltage=0  Measurements=None
  Three-Phase V-I Measurement : spsThreePhaseVIMeasurementLib/Three-Phase V-I Measurement  VoltageMeasurement=no  SetLabelV=off  LabelV=Vabc  Vpu=off  VpuLL=off  CurrentMeasurement=yes  SetLabelI=off  LabelI=Iabc  Ipu=off  Pbase=100e6  Vbase=500e3  OutputType=Complex  PhasorSimulation=off  PSBequivalent=0
  A : PMIOPort  Side=Left
  B : PMIOPort  Port=2  Side=Left
  C : PMIOPort  Port=3  Side=Left
  a : PMIOPort  Port=4  Side=Right
  b : PMIOPort  Port=5  Side=Right
  c : PMIOPort  Port=6  Side=Right
  i_abc : Outport
  wires:
  Three-Phase V-I Measurement/1 -> i_abc/1
  connections:
  Series RLC Branch/RConn1 -- Three-Phase V-I Measurement/LConn1
  Series RLC Branch1/RConn1 -- Three-Phase V-I Measurement/LConn2
  Series RLC Branch2/RConn1 -- Three-Phase V-I Measurement/LConn3
  A/RConn1 -- Series RLC Branch/LConn1
  a/RConn1 -- Three-Phase V-I Measurement/RConn1
  B/RConn1 -- Series RLC Branch1/LConn1
  b/RConn1 -- Three-Phase V-I Measurement/RConn2
  C/RConn1 -- Series RLC Branch2/LConn1
  c/RConn1 -- Three-Phase V-I Measurement/RConn3

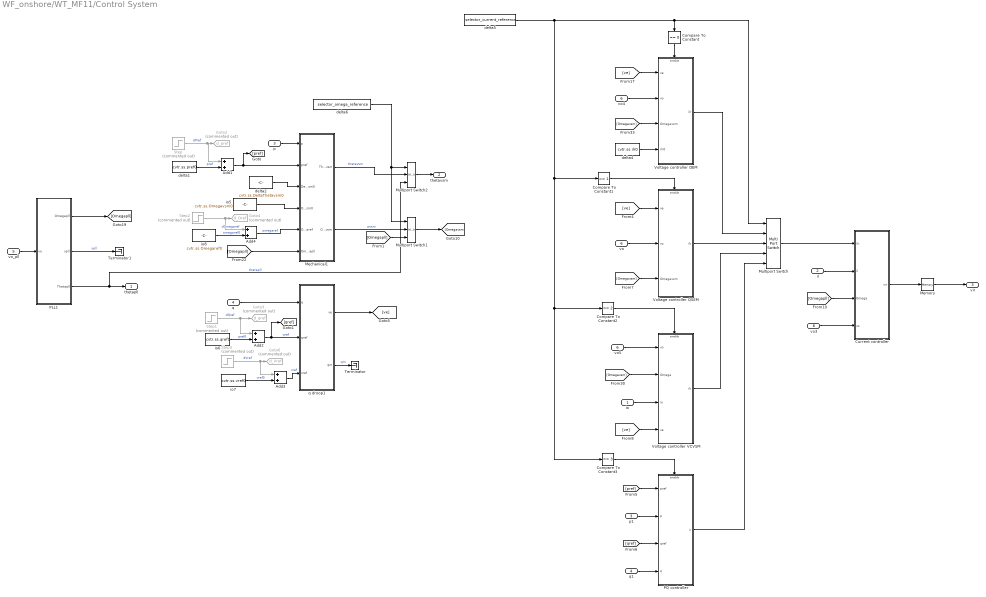
== system WF_onshore/WT_MF11/Control System ==
  io : Inport
  il : Inport  Port=2
  p : Inport  Port=3
  q : Inport  Port=4
  vo_pll : Inport  Port=5
  vo : Inport  Port=6
  Add{1..4} (4 alike) : Sum
  Compare To Constant : simulink/Logic and Bit Operations/Compare To Constant  relop===  const=0  OutDataTypeStr=boolean
  Compare To Constant1 : simulink/Logic and Bit Operations/Compare To Constant  relop===  const=1  OutDataTypeStr=boolean
  Compare To Constant2 : simulink/Logic and Bit Operations/Compare To Constant  relop===  const=2  OutDataTypeStr=boolean
  Compare To Constant3 : simulink/Logic and Bit Operations/Compare To Constant  relop===  const=3  OutDataTypeStr=boolean
  Current controller : Subsystem
  Goto2 : Goto  Commented=on  GotoTag=d_pref  TagVisibility=global
  Goto3 : Goto  Commented=on  GotoTag=d_qref  TagVisibility=global
  Goto4 : Goto  Commented=on  GotoTag=d_Oref  TagVisibility=global
  Goto6 : Goto  Commented=on  GotoTag=d_Vref  TagVisibility=global
  Mechanical1 : Subsystem
  Memory : Memory  InitialCondition=cvtr.ss.vir0
  Multiport Switch : MultiPortSwitch  DataPortOrder=Zero-based contiguous  Inputs=4  zeroidx=on  SaturateOnIntegerOverflow=off  InputSameDT=off
  Multiport Switch1 : MultiPortSwitch  DataPortOrder=Zero-based contiguous  Inputs=2  zeroidx=on  SaturateOnIntegerOverflow=off  InputSameDT=off
  Multiport Switch2 : MultiPortSwitch  DataPortOrder=Zero-based contiguous  Inputs=2  zeroidx=on  SaturateOnIntegerOverflow=off  InputSameDT=off
  PLL1 : Subsystem
  PQ controller : Subsystem
  Step : Step  Commented=on  After=0.01  SampleTime=0
  Step1 : Step  Commented=on  Time=1.5  After=0.03  SampleTime=0
  Step2 : Step  Commented=on  Time=2  After=0.001  SampleTime=0
  Step3 : Step  Commented=on  Time=2  After=0.001  SampleTime=0
  Terminator : Terminator
  Terminator1 : Terminator
  Voltage controller DEM : Subsystem
  Voltage controller QSEM : Subsystem
  Voltage controller VCVSM : Subsystem
  delta1 : Constant  Value=cvtr.ss.pref0
  delta2 : Constant  Value=cvtr.ss.DeltaThetavsm0
  delta4 : Constant  Value=cvtr.ss.ilr0
  delta5 : Constant  Value=selector_current_reference
  delta6 : Constant  Value=selector_omega_reference
  io5 : Constant  Value=cvtr.ss.Omegavsm0
  io6 : Constant  Value=cvtr.ss.qref0
  io7 : Constant  Value=cvtr.ss.vref0
  io8 : Constant  Value=cvtr.ss.Omegaref0
  p1 : InportShadow  Port=3
  q droop1 : Subsystem
  q1 : InportShadow  Port=4
  vo3 : InportShadow  Port=6
  vo4 : InportShadow  Port=6
  vo5 : InportShadow  Port=6
  thetapll : Outport
  thetavsm : Outport  Port=2
  vir : Outport  Port=3
  wires:
  io5/1 -> Mechanical1/4(Omegavsm0)
  Voltage controller DEM/1(ilr) -> Multiport Switch/2
  Add1/1 -> [pref], Mechanical1/2(pref)
  delta4/1 -> Voltage controller DEM/4(ilr0)
  Multiport Switch/1 -> Current controller/1(ilr)
  delta2/1 -> Mechanical1/3(DeltaThetavsm0)
  Add2/1 -> [qref], q droop1/2(qref)  "qref"
  delta1/1 -> Add1/2  "pref"
  q droop1/2(qm) -> Terminator/1  "qm"
  Add4/1 -> Mechanical1/5(Omegaref)  "omegaref"
  io7/1 -> Add3/2  "vref0"
  [Omegavsm] -> Voltage controller QSEM/3(Omegavsm)
  io8/1 -> Add4/2  "omegaref0"
  Step/1 -> Add1/1, Goto2/1  "dPref"
  [ve] -> Voltage controller QSEM/1(ve)
  delta5/1 -> Compare To Constant3/1, Compare To Constant2/1, Compare To Constant1/1, Multiport Switch/1, Compare To Constant/1
  io6/1 -> Add2/2  "qref0"
  Add3/1 -> q droop1/3(vref)  "vref"
  q/1 -> q droop1/1(q)
  [Omegavsm] -> Voltage controller VCVSM/2(Omega)
  [ve] -> Voltage controller DEM/1(ve)
  [Omegapll] -> Mechanical1/6(Omegapll)
  [Omegavsm] -> Voltage controller DEM/3(Omegavsm)
  p/1 -> Mechanical1/1(p)
  Voltage controller VCVSM/1(ilr) -> Multiport Switch/4
  vo/1 -> Voltage controller QSEM/2(vo)
  vo_pll/1 -> PLL1/1(vo)
  PLL1/2(vpll) -> Terminator1/1  "vpll"
  q droop1/1(ve) -> [ve]
  Voltage controller QSEM/1(ilr) -> Multiport Switch/3
  Memory/1 -> vir/1
  Current controller/1(vir) -> Memory/1
  p1/1 -> PQ controller/2(p)
  q1/1 -> PQ controller/4(q)
  PQ controller/1(ir) -> Multiport Switch/5
  il/1 -> Current controller/2(il)
  delta6/1 -> Multiport Switch2/1, Multiport Switch1/1
  [Omegapll] -> Current controller/3(Omega)
  Mechanical1/2(Omegavsm) -> Multiport Switch1/2  "wvsm"
  [Omegapll] -> Multiport Switch1/3
  Multiport Switch2/1 -> thetavsm/1
  Mechanical1/1(Thetavsm) -> Multiport Switch2/2  "thetavsm"
  Compare To Constant/1 -> Voltage controller DEM/Enable
  Compare To Constant1/1 -> Voltage controller QSEM/Enable
  Compare To Constant2/1 -> Voltage controller VCVSM/Enable
  Compare To Constant3/1 -> PQ controller/Enable
  Multiport Switch1/1 -> [Omegavsm]
  PLL1/1(Omegapll) -> [Omegapll]
  PLL1/3(Thetapll) -> Multiport Switch2/3, thetapll/1  "thetapll"
  io/1 -> Voltage controller VCVSM/3(io)
  vo3/1 -> Current controller/4(vo)
  vo4/1 -> Voltage controller DEM/2(vo)
  vo5/1 -> Voltage controller VCVSM/1(vo)
  [ve] -> Voltage controller VCVSM/4(ve)
  [pref] -> PQ controller/1(pref)
  [qref] -> PQ controller/3(qref)
  Step1/1 -> Goto3/1, Add2/1  "dQref"
  Step2/1 -> Add4/1, Goto4/1  "dOmegaref"
  Step3/1 -> Add3/1, Goto6/1  "dVref"

== system WF_onshore/WT_MF11/Inverse Park1 ==
  x_dq : Inport
  delta : Inport  Port=2
  Demux1 : Demux  Outputs=2
  Fcn : Fcn  Expr=cos(u(3))*u(1)-sin(u(3))*u(2)
  Fcn1 : Fcn  Expr=cos(u(3)-2/3*pi)*u(1)-sin(u(3)-2/3*pi)*u(2)
  Fcn2 : Fcn  Expr=cos(u(3)+2/3*pi)*u(1)-sin(u(3)+2/3*pi)*u(2)
  Mux : Mux  Inputs=3
  Mux1 : Mux  Inputs=3
  x_abc : Outport
  wires:
  Mux/1 -> Fcn1/1, Fcn2/1, Fcn/1
  Demux1/2 -> Mux/2
  Demux1/1 -> Mux/1
  Fcn/1 -> Mux1/1
  Fcn1/1 -> Mux1/2
  Fcn2/1 -> Mux1/3
  Mux1/1 -> x_abc/1
  x_dq/1 -> Demux1/1
  delta/1 -> Mux/3

== system WF_onshore/WT_MF11/Subsystem1 ==
  v_abc : Inport
  Controlled Voltage Source : spsControlledVoltageSourceLib/Controlled Voltage Source  Initialize=on  Source_Type=AC  Amplitude=0  Phase=0  Frequency=0  Measurements=None
  Controlled Voltage Source1 : spsControlledVoltageSourceLib/Controlled Voltage Source  Initialize=on  Source_Type=AC  Amplitude=0  Phase=0  Frequency=0  Measurements=None
  Controlled Voltage Source2 : spsControlledVoltageSourceLib/Controlled Voltage Source  Initialize=on  Source_Type=AC  Amplitude=0  Phase=0  Frequency=0  Measurements=None
  Demux : Demux  Outputs=3
  Ground : spsGroundLib/Ground  LConnTagsString=a
  va1 : PMIOPort  Side=Right
  vb1 : PMIOPort  Port=2  Side=Right
  vc1 : PMIOPort  Port=3  Side=Right
  wires:
  v_abc/1 -> Demux/1
  Demux/3 -> Controlled Voltage Source2/1
  Demux/2 -> Controlled Voltage Source1/1
  Demux/1 -> Controlled Voltage Source/1
  connections:
  Controlled Voltage Source/LConn1 -- Controlled Voltage Source1/LConn1 -- Controlled Voltage Source2/LConn1 -- Ground/LConn1
  vc1/RConn1 -- Controlled Voltage Source2/RConn1
  vb1/RConn1 -- Controlled Voltage Source1/RConn1
  va1/RConn1 -- Controlled Voltage Source/RConn1

== system WF_onshore/WT_MF11/Subsystem6 ==
  x_d+ix_q : Inport
  Complex to Real-Imag2 : ComplexToRealImag
  Mux : Mux  Inputs=2
  x_dq : Outport
  wires:
  Complex to Real-Imag2/1 -> Mux/1
  Complex to Real-Imag2/2 -> Mux/2
  Mux/1 -> x_dq/1
  x_d+ix_q/1 -> Complex to Real-Imag2/1

== system WF_onshore/WT_MF11/Transformations (pu and dq) ==
  i_abc_grid : Inport
  i_abc_filt : Inport  Port=2
  v_abc_grid : Inport  Port=3
  v_abc_filt : Inport  Port=4
  Thetavsm : Inport  Port=5
  Thetapll : Inport  Port=6
  3-phase Instantaneous Active & Reactive Power : powerlib_extras/Measurements/3-phase  Instantaneous  Active & Reactive Power
  Demux : Demux  Outputs=2
  Gain : Gain  Gain=1/cvtr.pu.Vb
  Gain1 : Gain  Gain=1/cvtr.pu.Ib
  Gain2 : Gain  Gain=1/cvtr.pu.Sb
  Gain4 : Gain  Gain=1/cvtr.pu.Ib
  Gain6 : Gain  Gain=1/cvtr.pu.Vb
  Park : Subsystem
  Park1 : Subsystem
  Park2 : Subsystem
  Park4 : Subsystem
  Subsystem2 : Subsystem
  Subsystem3 : Subsystem
  Subsystem4 : Subsystem
  Subsystem7 : Subsystem
  io : Outport
  il : Outport  Port=2
  p : Outport  Port=3
  q : Outport  Port=4
  vo_pll : Outport  Port=5
  vo : Outport  Port=6
  wires:
  Gain6/1 -> Park4/1(x_abc)
  i_abc_grid/1 -> 3-phase Instantaneous Active & Reactive Power/2, Gain1/1
  Gain2/1 -> Demux/1
  Gain1/1 -> Park1/1(x_abc)
  Gain/1 -> Park2/1(x_abc)
  Gain4/1 -> Park/1(x_abc)
  Park4/1(x_dq) -> Subsystem2/1(x_dq)
  Demux/1 -> p/1
  i_abc_filt/1 -> Gain4/1
  Thetapll/1 -> Park4/2(delta)
  Subsystem2/1(x_d+ix_q) -> vo_pll/1
  Thetavsm/1 -> Park1/2(delta), Park2/2(delta), Park/2(delta)
  Demux/2 -> q/1
  v_abc_grid/1 -> 3-phase Instantaneous Active & Reactive Power/1
  3-phase Instantaneous Active & Reactive Power/1 -> Gain2/1
  Subsystem4/1(x_d+ix_q) -> io/1
  Subsystem7/1(x_d+ix_q) -> il/1
  Subsystem3/1(x_d+ix_q) -> vo/1
  Park/1(x_dq) -> Subsystem7/1(x_dq)
  Park1/1(x_dq) -> Subsystem4/1(x_dq)
  Park2/1(x_dq) -> Subsystem3/1(x_dq)
  v_abc_filt/1 -> Gain/1, Gain6/1

== system WF_onshore/WT_MF11/filter capacitance1 ==
  Ground : spsGroundLib/Ground  LConnTagsString=a
  Series RLC Branch : spsSeriesRLCBranchLib/Series RLC Branch  LConnTagsString=__new0  RConnTagsString=__new0  BranchType=C  Resistance=R  Inductance=L  SetiL0=on  InitialCurrent=ia0  Capacitance=cvtr.parameters.Cf  Setx0=on  InitialVoltage=cvtr.ss.vo0a  Measurements=None
  Series RLC Branch1 : spsSeriesRLCBranchLib/Series RLC Branch  LConnTagsString=__new0  RConnTagsString=__new0  BranchType=C  Resistance=R  Inductance=L  SetiL0=on  InitialCurrent=ia0  Capacitance=cvtr.parameters.Cf  Setx0=on  InitialVoltage=cvtr.ss.vo0b  Measurements=None
  Series RLC Branch2 : spsSeriesRLCBranchLib/Series RLC Branch  LConnTagsString=__new0  RConnTagsString=__new0  BranchType=C  Resistance=R  Inductance=L  SetiL0=on  InitialCurrent=ia0  Capacitance=cvtr.parameters.Cf  Setx0=on  InitialVoltage=cvtr.ss.vo0c  Measurements=None
  Three-Phase V-I Measurement : spsThreePhaseVIMeasurementLib/Three-Phase V-I Measurement  VoltageMeasurement=phase-to-ground  SetLabelV=off  LabelV=Vabc  Vpu=off  VpuLL=off  CurrentMeasurement=no  SetLabelI=off  LabelI=Iabc  Ipu=off  Pbase=100e6  Vbase=500e3  OutputType=Complex  PhasorSimulation=off  PSBequivalent=0
  A : PMIOPort  Side=Left
  B : PMIOPort  Port=2  Side=Left
  C : PMIOPort  Port=3  Side=Left
  v_abc : Outport
  wires:
  Three-Phase V-I Measurement/1 -> v_abc/1
  connections:
  A/RConn1 -- Three-Phase V-I Measurement/LConn1
  B/RConn1 -- Three-Phase V-I Measurement/LConn2
  C/RConn1 -- Three-Phase V-I Measurement/LConn3
  Three-Phase V-I Measurement/RConn1 -- Series RLC Branch/LConn1
  Three-Phase V-I Measurement/RConn2 -- Series RLC Branch1/LConn1
  Three-Phase V-I Measurement/RConn3 -- Series RLC Branch2/LConn1
  Series RLC Branch/RConn1 -- Ground/LConn1 -- Series RLC Branch1/RConn1 -- Series RLC Branch2/RConn1

== system WF_onshore/WT_MF11/filter inductance1 ==
  Series RLC Branch : spsSeriesRLCBranchLib/Series RLC Branch  LConnTagsString=__new0  RConnTagsString=__new0  BranchType=RL  Resistance=cvtr.parameters.Rf  Inductance=cvtr.parameters.Lf  SetiL0=on  InitialCurrent=cvtr.ss.il0a  Capacitance=1e-6  Setx0=off  InitialVoltage=0  Measurements=None
  Series RLC Branch1 : spsSeriesRLCBranchLib/Series RLC Branch  LConnTagsString=__new0  RConnTagsString=__new0  BranchType=RL  Resistance=cvtr.parameters.Rf  Inductance=cvtr.parameters.Lf  SetiL0=on  InitialCurrent=cvtr.ss.il0b  Capacitance=1e-6  Setx0=off  InitialVoltage=0  Measurements=None
  Series RLC Branch2 : spsSeriesRLCBranchLib/Series RLC Branch  LConnTagsString=__new0  RConnTagsString=__new0  BranchType=RL  Resistance=cvtr.parameters.Rf  Inductance=cvtr.parameters.Lf  SetiL0=on  InitialCurrent=cvtr.ss.il0c  Capacitance=1e-6  Setx0=off  InitialVoltage=0  Measurements=None
  Three-Phase V-I Measurement : spsThreePhaseVIMeasurementLib/Three-Phase V-I Measurement  VoltageMeasurement=no  SetLabelV=off  LabelV=Vabc  Vpu=off  VpuLL=off  CurrentMeasurement=yes  SetLabelI=off  LabelI=Iabc  Ipu=off  Pbase=100e6  Vbase=500e3  OutputType=Complex  PhasorSimulation=off  PSBequivalent=0
  A : PMIOPort  Side=Left
  B : PMIOPort  Port=2  Side=Left
  C : PMIOPort  Port=3  Side=Left
  a : PMIOPort  Port=4  Side=Right
  b : PMIOPort  Port=5  Side=Right
  c : PMIOPort  Port=6  Side=Right
  i_abc : Outport
  wires:
  Three-Phase V-I Measurement/1 -> i_abc/1
  connections:
  c/RConn1 -- Three-Phase V-I Measurement/RConn3
  C/RConn1 -- Series RLC Branch2/LConn1
  b/RConn1 -- Three-Phase V-I Measurement/RConn2
  B/RConn1 -- Series RLC Branch1/LConn1
  a/RConn1 -- Three-Phase V-I Measurement/RConn1
  A/RConn1 -- Series RLC Branch/LConn1
  Series RLC Branch2/RConn1 -- Three-Phase V-I Measurement/LConn3
  Series RLC Branch1/RConn1 -- Three-Phase V-I Measurement/LConn2
  Series RLC Branch/RConn1 -- Three-Phase V-I Measurement/LConn1
